simulink model "Project"  (R2024a)
settings: Solver=VariableStepAuto  StartTime=0.0  StopTime=10.0  RelTol=1e-3
libraries: SignalEditorBlockLib x1
settings Model: Creator=mugiw  LastModifiedBy=mugiw

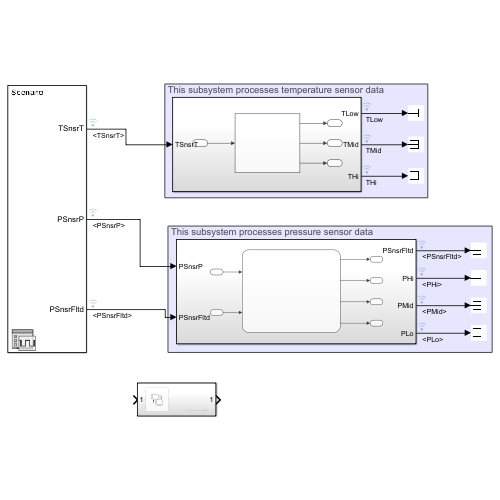
[thumbnail: Simulink's stored preview of the top-level diagram]
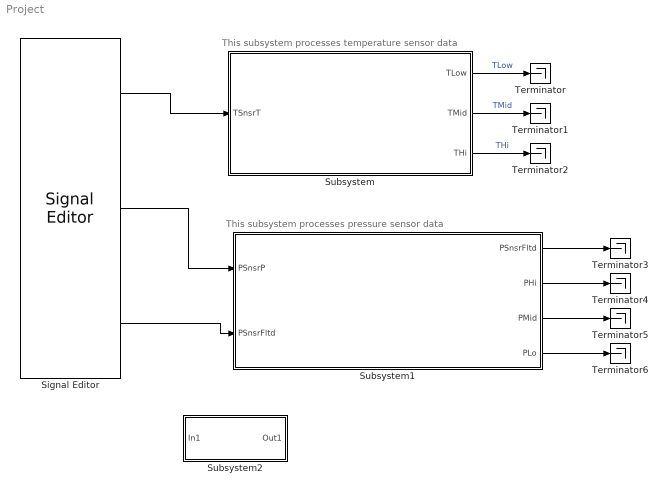
== system Project ==
  note: This subsystem processes pressure sensor data
  note: This subsystem processes temperature sensor data
  Signal Editor : SignalEditorBlockLib/Signal Editor  FileName=TempSignal.mat  ActiveScenario=Scenario  ActiveSignal=TSnsrT  IsBus=off  OutputBusObjectStr=Bus: BusObject  SampleTime=0  Interpolate=off  ZeroCross=off  OutputAfterFinalValue=Setting to zero  Unit=inherit  PreserveSignalName=on  ApplySigPropsToAllScenarios=on  ApplySigPropsToAllSignals=off
  Subsystem : Subsystem
  Subsystem1 : Subsystem
  Subsystem2 : Subsystem
  Terminator{,1..6} (7 alike) : Terminator
  wires:
  Subsystem/2(TMid) -> Terminator1/1  "TMid"
  Subsystem/3(THi) -> Terminator2/1  "THi"
  Subsystem/1(TLow) -> Terminator/1  "TLow"
  Subsystem1/1(PSnsrFltd) -> Terminator3/1
  Subsystem1/2(PHi) -> Terminator4/1
  Subsystem1/3(PMid) -> Terminator5/1
  Subsystem1/4(PLo) -> Terminator6/1
  Signal Editor/3 -> Subsystem1/2("PSnsrFltd ")
  Signal Editor/2 -> Subsystem1/1(PSnsrP)
  Signal Editor/1 -> Subsystem/1(TSnsrT)

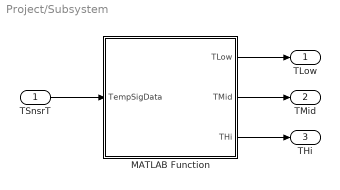
== system Project/Subsystem ==
  TSnsrT : Inport
  MATLAB Function : MATLAB Function  TreatAsAtomicUnit=on
  TLow : Outport
  TMid : Outport  Port=2
  THi : Outport  Port=3
  wires:
  TSnsrT/1 -> MATLAB Function/1(TempSigData)
  MATLAB Function/1(TLow) -> TLow/1
  MATLAB Function/2(TMid) -> TMid/1
  MATLAB Function/3(THi) -> THi/1

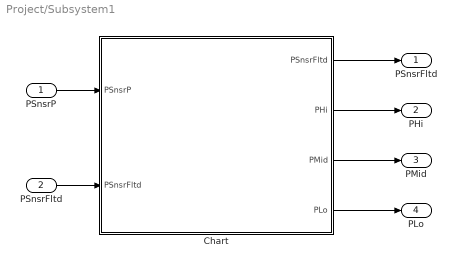
== system Project/Subsystem1 ==
  PSnsrP : Inport
  "PSnsrFltd " : Inport  Port=2
  Chart : Stateflow chart  TreatAsAtomicUnit=on
  PSnsrFltd : Outport
  PHi : Outport  Port=2
  PMid : Outport  Port=3
  PLo : Outport  Port=4
  wires:
  Chart/1(PSnsrFltd) -> PSnsrFltd/1
  Chart/2(PHi) -> PHi/1
  Chart/3(PMid) -> PMid/1
  Chart/4(PLo) -> PLo/1
  "PSnsrFltd "/1 -> Chart/2("PSnsrFltd ")
  PSnsrP/1 -> Chart/1(PSnsrP)

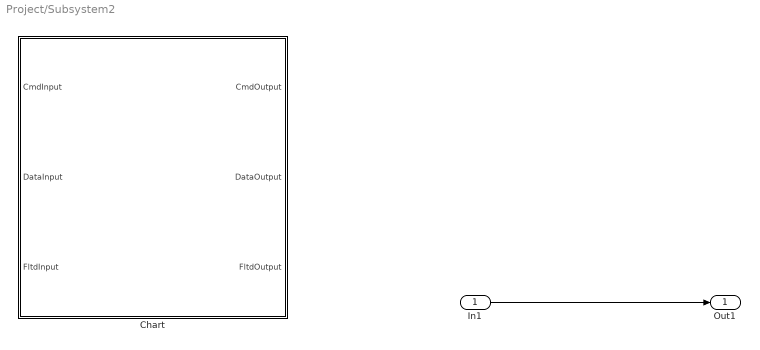
== system Project/Subsystem2 ==
  In1 : Inport
  Chart : Stateflow chart  TreatAsAtomicUnit=on
  Out1 : Outport
  wires:
  In1/1 -> Out1/1

== stateflow chart Project/Subsystem1/Chart ==
  (default) -> (junction 57) : {PHi = false;
      | PMid = false;
      | PLo = false;}
  (junction 57) -> (junction 58) [order 1] : [PSnsrFltd == true]
  (junction 57) -> (junction 59) [order 2]
  (junction 58) -> (junction 66)
  (junction 59) -> (junction 60) [order 1] : [PSnsrP <= 100]
  (junction 59) -> (junction 61) [order 2]
  (junction 60) -> (junction 65) : {PLo = true;}
  (junction 61) -> (junction 62) [order 1] : [PSnsrP <= 200]
  (junction 61) -> (junction 63) [order 2] : {PHi = true;}
  (junction 62) -> (junction 64) : {PMid = true;}
  (junction 64) -> (junction 63)
  (junction 65) -> (junction 64)
  (junction 66) -> (junction 65)
  (junction 63) -> (junction 67)
  data: PSnsrP input; PSnsrFltd input; PSnsrFltd output; PHi output; PMid output; PLo output

== stateflow chart Project/Subsystem2/Chart ==
  state Logic1
    entry:
    DataOutput = DataInput;
    CmdOutput = CmdInput;
    FltdOutput = FltdInput;
  state Logic2_3
    entry:
    DataOutput = 0;
    CmdOutput = false;
    FltdOutput = false;
  state Logic4
    entry,during:
    CmdOutput = false;
    FltdOutput = true;
    DataOutput = 0;
  Logic1 -> (junction 9)
  Logic2_3 -> (junction 9)
  (default) -> (junction 9)
  (junction 9) -> Logic1 [order 1] : [CmdInput && ~FltdInput]
  (junction 9) -> Logic2_3 [order 2] : [~CmdInput]
  (junction 9) -> Logic4 [order 3] : [CmdInput && FltdInput]
  Logic4 -> Logic2_3 : [~CmdInput]
  data: CmdInput input; DataInput input; FltdInput input; CmdOutput output; DataOutput output; FltdOutput output

== matlab function Project/Subsystem/MATLAB Function ==
  data: TempSigData input; TLow output; TMid output; THi output
function [TLow,TMid,THi] = fcn(TempSigData)

TLow = false;
TMid = false;
THi = false;

if(TempSigData <= 100)
    TLow = true;
elseif((TempSigData > 100) && (TempSigData <= 200))
    TMid = true;
else
    THi = true;
end
